simulink model "boatCtrlDemo"  (R2022b)
settings: Solver=FixedStepAuto  StartTime=0.0  StopTime=10  FixedStep=0.01  RelTol=1e-3
settings Model: Creator=71786  LastModifiedBy=71786
settings DataIOCC: ReturnWorkspaceOutputs=off

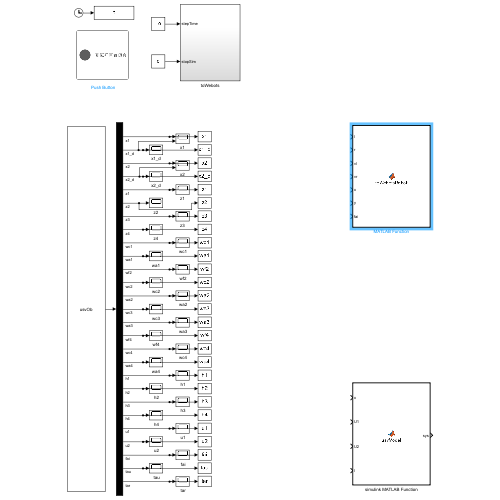
[thumbnail: Simulink's stored preview of the top-level diagram]
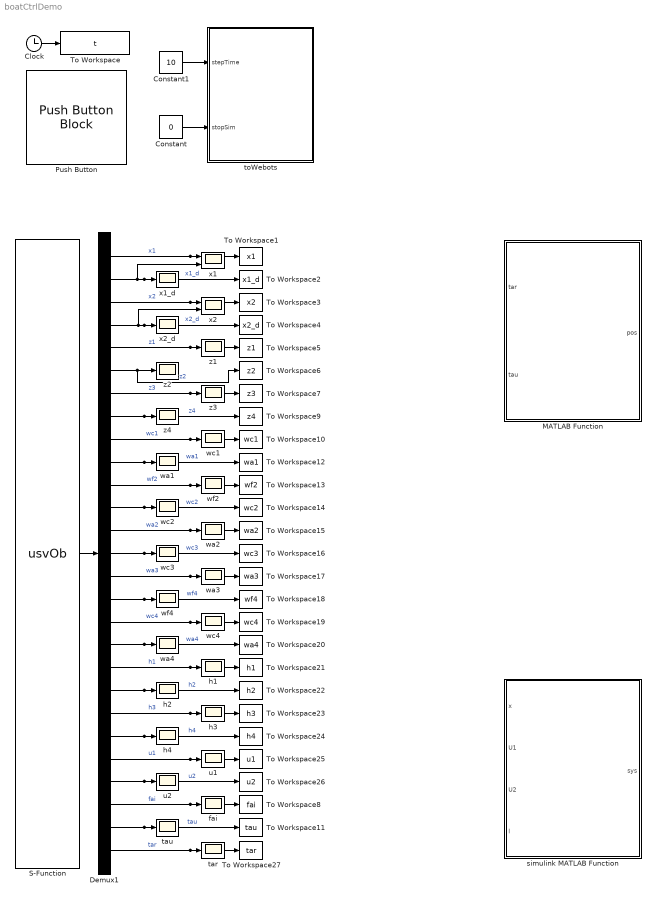
== system boatCtrlDemo ==
  " fai" : Scope
   h{1..4} (4 alike) : Scope
  " tar" : Scope
  " tau" : Scope
  " u1" : Scope
  " u2" : Scope
  " wa2" : Scope
  " wa3" : Scope
  " wc1" : Scope
  " wc4" : Scope
  " wf2" : Scope
  Clock : Clock
  Constant : Constant  Value=0
  Constant1 : Constant  Value=10
  Demux1 : Demux  Outputs=27
  MATLAB Function : MATLAB Function  TreatAsAtomicUnit=on
  Push Button : PushButtonBlock  ButtonText=复位并重置仿真  Icon=Circle  OffValue=0.000000
  S-Function : S-Function  FunctionName=usvOb  SFunctionDeploymentMode=off  EnableBusSupport=off
  To Workspace : ToWorkspace  VariableName=t  SaveFormat=Timeseries  SampleTime=-1
  To Workspace1 : ToWorkspace  VariableName=x1  SaveFormat=Timeseries  SampleTime=-1
  To Workspace10 : ToWorkspace  VariableName=wc1  SaveFormat=Timeseries  SampleTime=-1
  To Workspace11 : ToWorkspace  VariableName=tau  SaveFormat=Timeseries  SampleTime=-1
  To Workspace12 : ToWorkspace  VariableName=wa1  SaveFormat=Timeseries  SampleTime=-1
  To Workspace13 : ToWorkspace  VariableName=wf2  SaveFormat=Timeseries  SampleTime=-1
  To Workspace14 : ToWorkspace  VariableName=wc2  SaveFormat=Timeseries  SampleTime=-1
  To Workspace15 : ToWorkspace  VariableName=wa2  SaveFormat=Timeseries  SampleTime=-1
  To Workspace16 : ToWorkspace  VariableName=wc3  SaveFormat=Timeseries  SampleTime=-1
  To Workspace17 : ToWorkspace  VariableName=wa3  SaveFormat=Timeseries  SampleTime=-1
  To Workspace18 : ToWorkspace  VariableName=wf4  SaveFormat=Timeseries  SampleTime=-1
  To Workspace19 : ToWorkspace  VariableName=wc4  SaveFormat=Timeseries  SampleTime=-1
  To Workspace2 : ToWorkspace  VariableName=x1_d  SaveFormat=Timeseries  SampleTime=-1
  To Workspace20 : ToWorkspace  VariableName=wa4  SaveFormat=Timeseries  SampleTime=-1
  To Workspace21 : ToWorkspace  VariableName=h1  SaveFormat=Timeseries  SampleTime=-1
  To Workspace22 : ToWorkspace  VariableName=h2  SaveFormat=Timeseries  SampleTime=-1
  To Workspace23 : ToWorkspace  VariableName=h3  SaveFormat=Timeseries  SampleTime=-1
  To Workspace24 : ToWorkspace  VariableName=h4  SaveFormat=Timeseries  SampleTime=-1
  To Workspace25 : ToWorkspace  VariableName=u1  SaveFormat=Timeseries  SampleTime=-1
  To Workspace26 : ToWorkspace  VariableName=u2  SaveFormat=Timeseries  SampleTime=-1
  To Workspace27 : ToWorkspace  VariableName=tar  SaveFormat=Timeseries  SampleTime=-1
  To Workspace3 : ToWorkspace  VariableName=x2  SaveFormat=Timeseries  SampleTime=-1
  To Workspace4 : ToWorkspace  VariableName=x2_d  SaveFormat=Timeseries  SampleTime=-1
  To Workspace5 : ToWorkspace  VariableName=z1  SaveFormat=Timeseries  SampleTime=-1
  To Workspace6 : ToWorkspace  VariableName=z2  SaveFormat=Timeseries  SampleTime=-1
  To Workspace7 : ToWorkspace  VariableName=z3  SaveFormat=Timeseries  SampleTime=-1
  To Workspace8 : ToWorkspace  VariableName=fai  SaveFormat=Timeseries  SampleTime=-1
  To Workspace9 : ToWorkspace  VariableName=z4  SaveFormat=Timeseries  SampleTime=-1
  simulink MATLAB Function : MATLAB Function  TreatAsAtomicUnit=on
  toWebots : Subsystem
  wa1 : Scope
  wa4 : Scope
  wc2 : Scope
  wc3 : Scope
  wf4 : Scope
  x1 : Scope  NumInputPorts=2
  x1_d : Scope
  x2 : Scope  NumInputPorts=2
  x2_d : Scope
  z{1..4} (4 alike) : Scope
  wires:
  Constant/1 -> toWebots/2(stopSim)
  Constant1/1 -> toWebots/1(stepTime)
  Demux1/21 -> To Workspace23/1, " h3"/1  "h3"
  Demux1/23 -> To Workspace25/1, " u1"/1  "u1"
  Demux1/22 -> " h4"/1, To Workspace24/1  "h4"
  Demux1/24 -> " u2"/1, To Workspace26/1  "u2"
  Demux1/1 -> To Workspace1/1, x1/1  "x1"
  Demux1/18 -> wa4/1, To Workspace20/1  "wa4"
  Demux1/14 -> wc3/1, To Workspace16/1  "wc3"
  Demux1/17 -> To Workspace19/1, " wc4"/1  "wc4"
  Demux1/16 -> wf4/1, To Workspace18/1  "wf4"
  Demux1/19 -> To Workspace21/1, " h1"/1  "h1"
  Demux1/15 -> To Workspace17/1, " wa3"/1  "wa3"
  Demux1/8 -> z4/1, To Workspace9/1  "z4"
  Demux1/9 -> To Workspace10/1, " wc1"/1  "wc1"
  Demux1/6 -> z2/1, To Workspace6/1  "z2"
  Demux1/13 -> To Workspace15/1, " wa2"/1  "wa2"
  Demux1/12 -> To Workspace14/1, wc2/1  "wc2"
  Demux1/10 -> wa1/1, To Workspace12/1  "wa1"
  Clock/1 -> To Workspace/1
  Demux1/7 -> To Workspace7/1, z3/1  "z3"
  Demux1/20 -> " h2"/1, To Workspace22/1  "h2"
  Demux1/5 -> To Workspace5/1, z1/1  "z1"
  Demux1/3 -> To Workspace3/1, x2/1  "x2"
  Demux1/2 -> x1_d/1, To Workspace2/1, x1/2  "x1_d"
  Demux1/4 -> x2_d/1, To Workspace4/1, x2/2  "x2_d"
  Demux1/11 -> To Workspace13/1, " wf2"/1  "wf2"
  S-Function/1 -> Demux1/1
  Demux1/25 -> To Workspace8/1, " fai"/1  "fai"
  Demux1/26 -> " tau"/1, To Workspace11/1  "tau"
  Demux1/27 -> To Workspace27/1, " tar"/1  "tar"

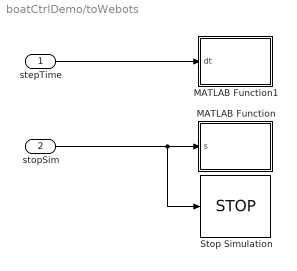
== system boatCtrlDemo/toWebots ==
  stepTime : Inport
  stopSim : Inport  Port=2
  MATLAB Function : MATLAB Function  TreatAsAtomicUnit=on
  MATLAB Function1 : MATLAB Function  TreatAsAtomicUnit=on
  Stop Simulation : Stop
  wires:
  stopSim/1 -> Stop Simulation/1, MATLAB Function/1(s)
  stepTime/1 -> MATLAB Function1/1(dt)

== matlab function boatCtrlDemo/toWebots/MATLAB Function ==
  data: s input
function resetSim(s)
    if s >= 1
        wb_supervisor_simulation_reset();
    end

== matlab function boatCtrlDemo/MATLAB Function ==
  data: tar input; tau input; pos output
function pos = toWebotsRobot(tar, tau)

end

== matlab function boatCtrlDemo/toWebots/MATLAB Function1 ==
  data: dt input
function robotStep(dt)
    wb_robot_step(dt);

== matlab function boatCtrlDemo/simulink MATLAB Function ==
  data: x input; U1 input; U2 input; l input; sys output
function sys  = usvModel(x, U1, U2, l)
    % usvModel - Unmanned Surface Vehicle dynamics model
    %
    % Inputs:
    %   x - State vector [X; Y; Phi; Vu; Vv; Vr; X1; X1_dot; Y1; Y1_dot]
    %   U1, U2 - Control inputs 
    %   l - Look-ahead distance parameter
    %
    % Outputs:
    %   sys - System derivatives (length 10 vector)
    %   Tau - Calculated thrust
    %   Tar - Calculated torque
    
    % Initialize output vector
    sys = zeros(10, 1);
    
    % System parameters
    m = [25.80 0 0;
         0 33.80 0;
         0 0 2.76];
    d = [0.72253 1.32742 0.008950;
         0.88965 36.4728 0.029575;
         1.90000 0.75000 0.007700];
    
    % Extract state variables
    Vu = x(4);
    Vv = x(5);
    Vr = x(6);
    Phi = x(3);
    
    % Calculate control forces
    Tau = (m(1,1)*(U1*cos(Phi)+U2*sin(Phi)))/(cos(Phi)^2+sin(Phi)^2);
    Tar = (m(3,3)*(cos(Phi)*U2-sin(Phi)*U1))/(l*(cos(Phi)^2+sin(Phi)^2));
    
    % Uncomment for saturation if needed
    % Tau_max = 10000;
    % Tar_max = 10000;
    % Tau = max(min(Tau, Tau_max), -Tau_max);
    % Tar = max(min(Tar, Tar_max), -Tar_max);
    
    % Original model equations
    sys(1) = Vu * cos(Phi) - Vv * sin(Phi);                         % dotX
    sys(2) = Vu * sin(Phi) + Vv * cos(Phi);                         % dotY
    sys(3) = Vr;                                                    % dotPhi
    sys(4) = (m(2,2)*Vv*Vr - d(1,1)*Vu + Tau)/m(1,1);               % dotVu
    sys(5) = (-m(1,1)*Vu*Vr - d(2,2)*Vv)/m(2,2);                    % dotVv
    sys(6) = ((m(1,1)-m(2,2))*Vu*Vv - d(3,3)*Vr + Tar)/m(3,3);      % dotVr
    
    % Unknown dynamics terms
    Fuv = (m(2,2)*Vv*Vr - d(1,1)*Vu)/m(1,1);                        % 未知动力学
    Fvv = (-m(1,1)*Vu*Vr - d(2,2)*Vv)/m(2,2);                       % 未知动力学
    Frv = ((m(1,1)-m(2,2))*Vu*Vv - d(3,3)*Vr)/m(3,3);               % 未知动力学
    
    % Transformed model equations 
    sys(7) = x(8);                                                  % 变换后 dotX1
    sys(8) = Fuv*cos(Phi)-(Fvv+l*Frv)*sin(Phi)-(Vu*Vr*sin(Phi)+(Vv*Vr+l*Vr^2)*cos(Phi)) ...
        + cos(Phi)/m(1,1)*Tau - l*sin(Phi)*Tar/m(3,3);              % 变换后 dot(dotX1)
    sys(9) = x(10);                                                 % 变换后 dotY1
    sys(10) = Fuv*sin(Phi)-(Fvv+l*Frv)*cos(Phi)+(Vu*Vr*cos(Phi)-(Vv*Vr+l*Vr^2)*sin(Phi)) ...
        + sin(Phi)/m(1,1)*Tau + l*cos(Phi)*Tar/m(3,3);              % 变换后 dot(dotY1)
end
